simulink model "MTU_HVM_5_0a"  (Simulink 7.7)
settings: Solver=ode23  StartTime=0.0  StopTime=TEST_CYCLE(end,1)  FixedStep=0.01  RelTol=1e-3
InitFcn:
  | Vehicle_Init_File
values from neighbouring files (symbols this model uses):
  Batt_Aux_Load_W = 800    [Student_Design_Parameters.m]
  Engine_ACC_Loss_Nm = 4.6    [ICE_Tech_Specs.m]
  Engine_BSFC_2DMAP_g_kWh = Engine_BSFC_2DMAP_g_kWh'    [ICE_Tech_Specs.m]    (also in Student_Design_Parameters.m = 1.00*Engine_BSFC_2DMAP_g_kWh)
  Engine_Max_Speed_rpm = 6800    [ICE_Tech_Specs.m]
  Engine_Min_Speed_rpm = 600    [ICE_Tech_Specs.m]
  Engine_Startup_Fuel_g = 4.0*Engine_Displacement_L/3.6    (= 2.66666666667)    [ICE_Tech_Specs.m]
  Engine_Torque_2DMAP_Nm = Engine_Torque_2DMAP_Nm'    [ICE_Tech_Specs.m]
  Motor_Gear_Ratio = 1.00    (= 1)    [Student_Design_Parameters.m]
  Motor_Km = 0.94    [Motor_Tech_Specs.m]
  Motor_Ra = 0.106    [Motor_Tech_Specs.m]
  Motor_Torque_Peak_Nm = T    [Motor_Tech_Specs.m]
  Motor_Torque_Speed_Index_rpm = N    [Motor_Tech_Specs.m]
  TEST_CYCLE = [0 1 2 3 4 5 6 7 8 9 10 11 ... (1900 elements, 950x2)]    [Constant_Speed_Points_Cycle.mat]    (also in US06_Cycle.mat = [0 1 2 3 4 5 6 7 8 9 10 11 ... (1202 elements, 601x2)])
  TRANS_Differential_Ratio = 3.25    [Student_Design_Parameters.m]
  TRANS_DS_THRES = 1.0*TRANS_DS_THRES    [Student_Design_Parameters.m]
  TRANS_US_THRES = 1.0*TRANS_US_THRES    [Student_Design_Parameters.m]
  Vehicle_Drag_Coeff = F2/(0.5*Air_Density_kgm*Vehicle_Frontal_Area_m)    [Student_Design_Parameters.m]
  Vehicle_Frontal_Area_m = h*w*0.0254*0.0254    [Student_Design_Parameters.m]
  Vehicle_Mass_kg = 1549    [Student_Design_Parameters.m]
  Vehicle_Tire_Coeff_Rolling_Resistance = 0.008    [Student_Design_Parameters.m]
  Vehicle_Tire_Radius_m = 0.95*26.311/2*0.0254    (= 0.317442215)    [Student_Design_Parameters.m]
undefined symbols (not defined in the file or in its folder): Air_Density_kgm, Batt_a, Batt_Capacity_Ah, Batt_Const_V, Batt_dG, Batt_Disable_SOC, Batt_Initial_SOC, Batt_Lower_Volt_Limit_V, Batt_Max_Charge_Current_A, Batt_Max_Discharge_Current_A, Batt_Max_SOC, Batt_Min_SOC, Batt_Numb_Cells_N, Batt_OCV_Z, Batt_Resis_Ohms, Batt_Upper_Volt_Limit_V, Batt_Warburg_Capcitance_F, Batt_Warburg_Resis_Ohms, Fuel_Density_kgm3, Gravity, Max_Vehicle_Speed_Control_Error_mph, TRANS_Gear_Ratio, Vehicle_Tire_Rolling_Fric_Velocity_Modifier, Vehicle_Tire_Static_Fric_Coeff, Vehicle_Tractive_Force_Limit
libraries: simulink x8
(part 1 of 2)
settings Model: Creator=lawyerkm  LastModifiedBy=jnaber
settings SolverCC: ZeroCrossControl=DisableAll
settings OptimizationCC: InitFltsAndDblsToZero=on
settings DebuggingCC: AlgebraicLoopMsg=none  ArtificialAlgebraicLoopMsg=none  SaveWithParameterizedLinksMsg=none  SolverPrmCheckMsg=none  InheritedTsInSrcMsg=none  DiscreteInheritContinuousMsg=none  MultiTaskCondExecSysMsg=none  UnknownTsInhSupMsg=none  StrictBusMsg=None
settings HardwareCC: TargetHWDeviceType=32-bit Generic
settings SFSimCC: SimParseCustomCode=off
settings RTWCC: IncludeERTFirstTime=on
settings GRTTargetCC: TargetFcnLib=ansi_tfl_tmw.mat

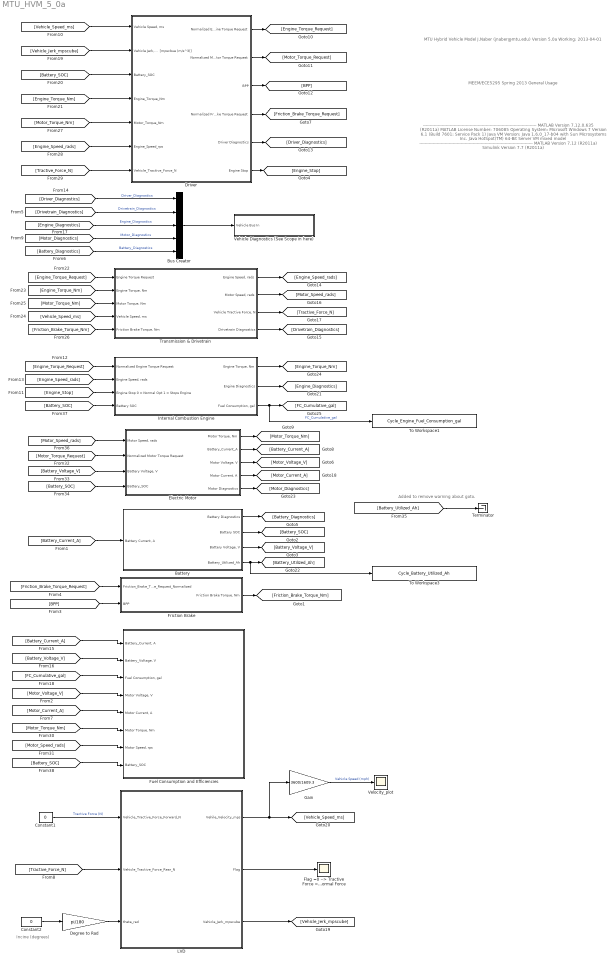
== system MTU_HVM_5_0a ==
  note: MTU Hybrid Vehicle Model
      | J.Naber (jnaber@mtu.edu)
      | Version 5.0a
      | Working:  2013-04-01
  note: MEEM/ECE5295
      | Spring 2013
      |
      | General Usage
  note: -------------------------------------------------------------------------------------
      | MATLAB Version 7.12.0.635 (R2011a)
      | MATLAB License Number: 706085
      | Operating System: Microsoft Windows 7 Version 6.1 (Build 7601: Service Pack 1)
      | Java VM Version: Java 1.6.0_17-b04 with Sun Microsystems Inc. Java HotSpot(TM) 64-Bit Server VM mixed model
      | -------------------------------------------------------------------------------------
      | MATLAB                                                Version 7.12       (R2011a)
      | Simulink                                                 Version 7.7        (R2011a)
  note: Added to remove warning about goto.
  note: Incine (degrees)
  Battery : Subsystem
  Bus Creator : BusCreator  Inputs=5
  Constant1 : Constant  Value=0
  Constant2 : Constant  Value=0
  Degree to Rad : Gain  Gain=pi/180
  Driver : Subsystem
  Electric Motor : Subsystem
  Flag =0 --> Tractive Force =< Road Friction * Normal Force Flag =1 --> Tractive Force > Road Friction * Normal Force : Scope
      settings: TimeRange=200  YMin=-1  YMax=1  SaveName=ScopeData2  SampleInput=on  SampleTime=0.5
  Friction Brake : Subsystem
  Fuel Consumption and Efficiencies : Subsystem
  Gain : Gain  Gain=3600/1609.3
  Internal Combustion Engine : Subsystem
  LVD : Subsystem
      mask help:
      | Vehicle of two axles riding on an incline. The aerodynamic parameters include the vehicle's frontal area and drag coefficient. The vehicle does not pitch or move vertically.
      |
      | The input signals Vehicle_Tractive_Force_Forward_N, Vehicle_Tractive_Force_Rear_N, and theta_rad specify the tractive force at forward and rear contact forces (N) and the incline angle (rad), respectively. The output signal Vehile_Velocity_mps, indicates the vehicle velocity (m/s).
      mask init:
      | g = 9.81;
      | rho = 1.2; %Air Density in kg/m^3
      mask Display:
      | port_label('input', 1, 'Vehicle_Tractive_Force_Front_N')
      | port_label('input', 2, 'Vehicle_Tractive_Force_Rear_N')
      | port_label('input', 3, 'theta_rad')
      | port_label('output', 1, 'Vehile_Velocity_mps')
      | port_label('output', 2, 'Flag')
      | port_label('output', 3, 'Vehicle_Jerk_mpscube')
  Terminator : Terminator
  To Workspace1 : ToWorkspace  VariableName=Cycle_Engine_Fuel_Consumption_gal  SampleTime=-1  SaveFormat=Array
      settings: MaxDataPoints=1
  To Workspace3 : ToWorkspace  VariableName=Cycle_Battery_Utilized_Ah  SampleTime=-1  SaveFormat=Array
      settings: MaxDataPoints=1
  Transmission & Drivetrain : Subsystem
  Vehicle Diagnostics (See Scope in here) : Subsystem
  Velocity_plot : Scope
      settings: TimeRange=200  YMax=60  SaveName=Vehicle_Speed  SampleTime=0.5
  wires:
  Driver/2(Normalized Motor Torque Request) -> [Motor_Torque_Request]
  Driver/1(Normalized Engine Torque Request) -> [Engine_Torque_Request]
  Driver/3(BPP) -> [BPP]
  Driver/5(Driver Diagnostics) -> [Driver_Diagnostics]
  [Vehicle_Speed_ms] -> Driver/1("Vehicle Speed, ms")
  [Driver_Diagnostics] -> Bus Creator/1  "Driver_Diagnostics"
  [Drivetrain_Diagnostics] -> Bus Creator/2  "Drivetrain_Diagnostics"
  Bus Creator/1 -> Vehicle Diagnostics (See Scope in here)/1(Vehicle Bus In)
  [Motor_Diagnostics] -> Bus Creator/4  "Motor_Diagnostics"
  [Battery_Diagnostics] -> Bus Creator/5  "Battery_Diagnostics"
  [Engine_Diagnostics] -> Bus Creator/3  "Engine_Diagnostics"
  LVD/1(Vehile_Velocity_mps) -> Gain/1, [Vehicle_Speed_ms]
  Constant1/1 -> LVD/1(Vehicle_Tractive_Force_Forward_N)  "Tractive Force (N)"
  Constant2/1 -> Degree to Rad/1
  Gain/1 -> Velocity_plot/1  "Vehicle Speed (mph)"
  LVD/2(Flag) -> Flag =0 --> Tractive Force =< Road Friction * Normal Force Flag =1 --> Tractive Force > Road Friction * Normal Force/1
  [Tractive_Force_N] -> LVD/2(Vehicle_Tractive_Force_Rear_N)
  [Battery_Current_A] -> Fuel Consumption and Efficiencies/1("Battery_Current, A")
  [FC_Cumulative_gal] -> Fuel Consumption and Efficiencies/3("Fuel Consumption, gal")
  [Battery_Voltage_V] -> Fuel Consumption and Efficiencies/2("Battery_Voltage, V")
  [Motor_Voltage_V] -> Fuel Consumption and Efficiencies/4("Motor Voltage, V")
  [Motor_Current_A] -> Fuel Consumption and Efficiencies/5("Motor Current, A")
  [Motor_Torque_Nm] -> Fuel Consumption and Efficiencies/6("Motor Torque, Nm")
  [Motor_Speed_rads] -> Fuel Consumption and Efficiencies/7("Motor Speed, rps")
  Transmission & Drivetrain/4(Drivetrain Diagnostics) -> [Drivetrain_Diagnostics]
  Transmission & Drivetrain/1("Engine Speed, rads") -> [Engine_Speed_rads]
  Transmission & Drivetrain/2("Motor Speed, rads") -> [Motor_Speed_rads]
  Transmission & Drivetrain/3("Vehicle Tractive Force, N") -> [Tractive_Force_N]
  [Engine_Torque_Request] -> Transmission & Drivetrain/1(Engine Torque Request)
  [Engine_Torque_Nm] -> Transmission & Drivetrain/2("Engine Torque, Nm")
  [Motor_Torque_Nm] -> Transmission & Drivetrain/3("Motor Torque, Nm")
  [Vehicle_Speed_ms] -> Transmission & Drivetrain/4("Vehicle Speed, ms")
  [Friction_Brake_Torque_Nm] -> Transmission & Drivetrain/5("Friction Brake Torque, Nm")
  [Motor_Speed_rads] -> Electric Motor/1("Motor Speed, rads")
  [Motor_Torque_Request] -> Electric Motor/2(Normalized Motor Torque Request)
  [Battery_Voltage_V] -> Electric Motor/3("Battery Voltage, V")
  Electric Motor/1("Motor Torque, Nm") -> [Motor_Torque_Nm]
  [Battery_SOC] -> Electric Motor/4(Battery_SOC)
  Driver/4(Normalized Friction Brake Torque Request) -> [Friction_Brake_Torque_Request]
  [BPP] -> Friction Brake/2(BPP)
  [Friction_Brake_Torque_Request] -> Friction Brake/1(Friction_Brake_Torque_Request_Normalized)
  Friction Brake/1("Friction Brake Torque, Nm") -> [Friction_Brake_Torque_Nm]
  Electric Motor/2(Battery_Current_A) -> [Battery_Current_A]
  Electric Motor/3("Motor Voltage, V") -> [Motor_Voltage_V]
  Electric Motor/4("Motor Current, A") -> [Motor_Current_A]
  Internal Combustion Engine/2(Engine Diagnostics) -> [Engine_Diagnostics]
  Internal Combustion Engine/1("Engine Torque, Nm") -> [Engine_Torque_Nm]
  [Engine_Torque_Request] -> Internal Combustion Engine/1(Normalized Engine Torque Request)
  [Engine_Speed_rads] -> Internal Combustion Engine/2("Engine Speed, rads")
  Internal Combustion Engine/3("Fuel Consumption, gal") -> [FC_Cumulative_gal], To Workspace1/1  "FC_Cumulative_gal"
  [Engine_Stop] -> Internal Combustion Engine/3(Engine Stop 0 = Normal Opt 1 = Stops Engine)
  Driver/6(Engine Stop) -> [Engine_Stop]
  LVD/3(Vehicle_Jerk_mpscube) -> [Vehicle_Jerk_mpscube]
  [Vehicle_Jerk_mpscube] -> Driver/2("Vehicle Jerk,  [mpscbue (m/s^3)]")
  Electric Motor/5(Motor Diagnostics) -> [Motor_Diagnostics]
  [Battery_SOC] -> Driver/3(Battery_SOC)
  [Engine_Torque_Nm] -> Driver/4(Engine_Torque_Nm)
  [Motor_Torque_Nm] -> Driver/5(Motor_Torque_Nm)
  [Engine_Speed_rads] -> Driver/6(Engine_Speed_rps)
  [Tractive_Force_N] -> Driver/7(Vehicle_Tractive_Force_N)
  [Battery_Utilized_Ah] -> Terminator/1
  [Battery_Current_A] -> Battery/1("Battery Current, A")
  Battery/1(Battery Diagnostics) -> [Battery_Diagnostics]
  [Battery_SOC] -> Internal Combustion Engine/4(Battery SOC)
  Battery/3("Battery Voltage, V") -> [Battery_Voltage_V]
  Battery/2(Battery SOC) -> [Battery_SOC]
  Battery/4(Battery_Utilized_Ah) -> [Battery_Utilized_Ah], To Workspace3/1
  [Battery_SOC] -> Fuel Consumption and Efficiencies/8("Battery_SOC ")
  Degree to Rad/1 -> LVD/3(theta_rad)

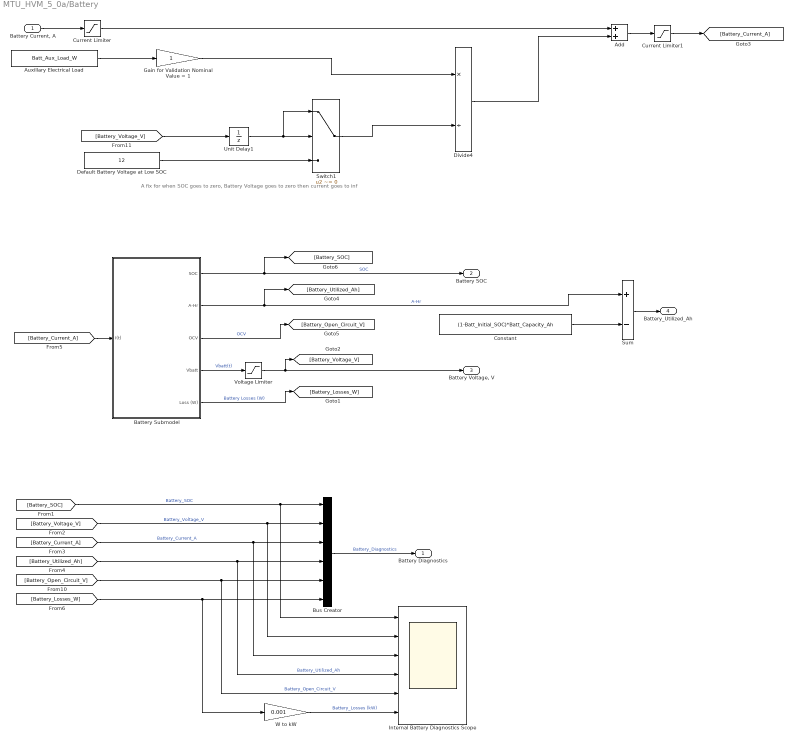
== system MTU_HVM_5_0a/Battery ==
  note: A fix for when SOC goes to zero,
      |  Battery Voltage goes to zero then current goes to inf
  "Battery Current, A" : Inport
  Add : Sum
  Auxillary Electrical Load : Constant  Value=Batt_Aux_Load_W
  Battery Submodel : Subsystem  mask{Vo=Batt_Const_V, Rbatt=Batt_Resis_Ohms, Cd=Batt_Warburg_Capcitance_F, Rd=Batt_Warburg_Resis_Ohms, Q=Batt_Capacity_Ah, dG=Batt_dG, a=Batt_a, SOC_Init=Batt_Initial_SOC, Batt_Numb_Cells_N=Batt_Numb_Cells_N, Batt_OCV_Z=Batt_OCV_Z}
      mask prompts: Vo "Fully Charged Voltage Vo (V)"; Rbatt "Battery Resistance Rc (Ohm)"; Cd "Warburg Capacitance Cd (F)"; Rd "Warburg Resistance Rd (Ohm)"; Q "Amp Hour Capacity  Q (A-Hr)"; dG "Free energy difference dG"; a "Molecular interaction exponent a"; SOC_Init "State of Charge Initial (-)"; Batt_Numb_Cells_N "Number of Cells"; Batt_OCV_Z "Z Parameter"
      mask help:
      | Lithium Cobalt Oxide/Carbon
      |     dG = -355000,   a = 4
      |
      | Nickel Metal Hydride
      |     dG = -115000,   a=0.8
  Bus Creator : BusCreator  Inputs=6
  Constant : Constant  Value=(1-Batt_Initial_SOC)*Batt_Capacity_Ah  SampleTime=-1
  Current Limiter : Saturate  UpperLimit=Batt_Max_Charge_Current_A  LowerLimit=Batt_Max_Discharge_Current_A
  Current Limiter1 : Saturate  UpperLimit=Batt_Max_Charge_Current_A  LowerLimit=Batt_Max_Discharge_Current_A
  Default Battery Voltage at Low SOC : Constant  Value=12  SampleTime=-1
  Divide4 : Product  Inputs=*/
  Gain for Validation Nominal Value = 1 : Gain
  Internal Battery Diagnostics Scope : Scope  NumInputPorts=6
      settings: TimeRange=1000  YMin=5.55112e-017~62.75~71.25~0.5~90~2.75  YMax=0.8~64.25~78.75~5~102~4.25  SaveName=Diagnostics_Battery  SampleInput=on  SampleTime=0.1
  Sum : Sum  Inputs=+-
  Switch1 : Switch  Criteria=u2 ~= 0  Threshold=12
  Unit Delay1 : UnitDelay  X0=Batt_Const_V  SampleTime=-1
  Voltage Limiter : Saturate  UpperLimit=Batt_Upper_Volt_Limit_V  LowerLimit=Batt_Lower_Volt_Limit_V  LinearizeAsGain=off
  W to kW : Gain  Gain=0.001
  Battery Diagnostics : Outport
  Battery SOC : Outport  Port=2
  "Battery Voltage, V" : Outport  Port=3
  Battery_Utilized_Ah : Outport  Port=4
  wires:
  Bus Creator/1 -> Battery Diagnostics/1  "Battery_Diagnostics"
  [Battery_SOC] -> Bus Creator/1, Internal Battery Diagnostics Scope/1  "Battery_SOC"
  [Battery_Voltage_V] -> Bus Creator/2, Internal Battery Diagnostics Scope/2  "Battery_Voltage_V"
  [Battery_Current_A] -> Bus Creator/3, Internal Battery Diagnostics Scope/3  "Battery_Current_A"
  "Battery Current, A"/1 -> Current Limiter/1
  [Battery_Utilized_Ah] -> Bus Creator/4, Internal Battery Diagnostics Scope/4  "Battery_Utilized_Ah"
  [Battery_Open_Circuit_V] -> Bus Creator/5, Internal Battery Diagnostics Scope/5  "Battery_Open_Circuit_V"
  Add/1 -> Current Limiter1/1
  Auxillary Electrical Load/1 -> Gain for Validation Nominal Value = 1/1
  [Battery_Losses_W] -> Bus Creator/6, W to kW/1
  Default Battery Voltage at Low SOC/1 -> Switch1/3
  [Battery_Voltage_V] -> Unit Delay1/1
  W to kW/1 -> Internal Battery Diagnostics Scope/6  "Battery_Losses (kW)"
  Switch1/1 -> Divide4/2
  Unit Delay1/1 -> Switch1/1, Switch1/2
  Battery Submodel/1(SOC) -> [Battery_SOC], Battery SOC/1  "SOC"
  Battery Submodel/2(A-Hr) -> [Battery_Utilized_Ah], Sum/1  "A-Hr"
  Battery Submodel/3(OCV) -> [Battery_Open_Circuit_V]  "OCV"
  Battery Submodel/5(Loss (W)) -> [Battery_Losses_W]  "Battery Losses (W)"
  Battery Submodel/4(Vbatt) -> Voltage Limiter/1  "Vbatt(t)"
  [Battery_Current_A] -> Battery Submodel/1(I(t))
  Divide4/1 -> Add/2
  Gain for Validation Nominal Value = 1/1 -> Divide4/1
  Current Limiter1/1 -> [Battery_Current_A]
  Current Limiter/1 -> Add/1
  Voltage Limiter/1 -> [Battery_Voltage_V], "Battery Voltage, V"/1
  Sum/1 -> Battery_Utilized_Ah/1
  Constant/1 -> Sum/2

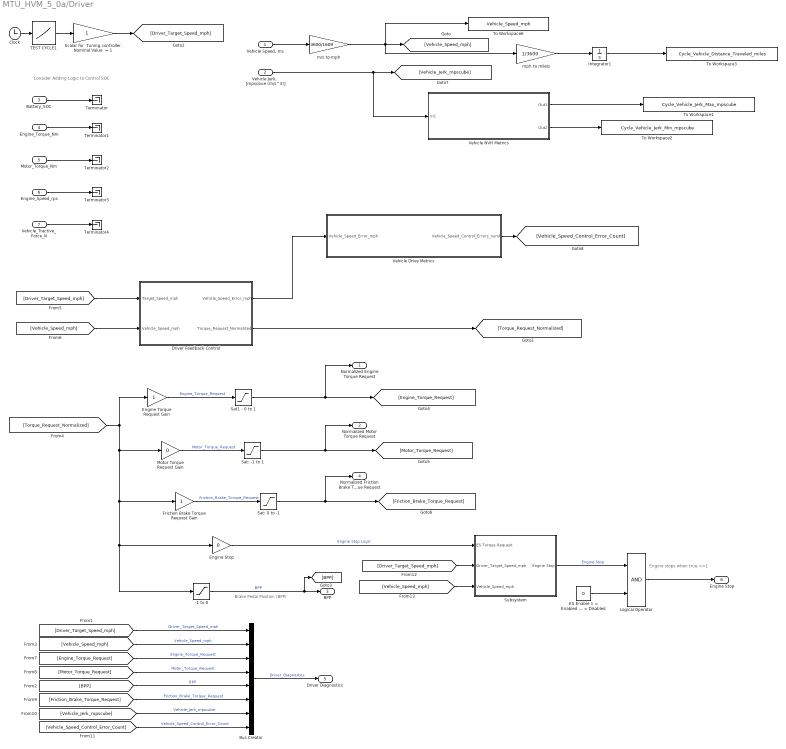
== system MTU_HVM_5_0a/Driver ==
  note: Consider Adding Logic to Control SOC
  note: Brake Pedal Position
      |
      | (BPP)
  note: Engine stops when
      |
      | true ==1
  "Vehicle Speed, ms" : Inport
  "Vehicle Jerk,  [mpscbue (m/s^3)]" : Inport  Port=2
  Battery_SOC : Inport  Port=3
  Engine_Torque_Nm : Inport  Port=4
  Motor_Torque_Nm : Inport  Port=5
  Engine_Speed_rps : Inport  Port=6
  Vehicle_Tractive_Force_N : Inport  Port=7
  -1 to 0 : Saturate  UpperLimit=0  LowerLimit=-1
  Bus Creator : BusCreator  Inputs=8
  Clock : Clock
      settings: Decimation=10
  Driver Feedback Control : Subsystem
  ES Enable 1 = Enabled 0 = Disabled : Constant  Value=0  SampleTime=-1
  "Engine Stop " : Gain  Gain=0
  Engine Torque Request Gain : Gain
  Friction Brake Torque Request Gain : Gain
  Integrator1 : Integrator
  Logical Operator : Logic  AllPortsSameDT=off  OutDataTypeStr=boolean
  Motor Torque Request Gain : Gain  Gain=0
  Sat1 - 0 to 1 : Saturate  UpperLimit=1  LowerLimit=0
  Sat: -1 to 1 : Saturate  UpperLimit=1  LowerLimit=-1
  Sat: 0 to -1 : Saturate  UpperLimit=0  LowerLimit=-1
  Scalar for  Tuning controller. Nominal Value  = 1 : Gain
  Subsystem : Subsystem
  TEST CYCLE1 : Lookup  InputValues=TEST_CYCLE(:,1)  Table=TEST_CYCLE(:,2)  LookUpMeth=Interpolation-Use End Values
  Terminator{,1..4} (5 alike) : Terminator
  To Workspace1 : ToWorkspace  VariableName=Cycle_Vehicle_Jerk_Max_mpscube  SampleTime=-1  SaveFormat=Array
      settings: MaxDataPoints=1
  To Workspace2 : ToWorkspace  VariableName=Cycle_Vehicle_Jerk_Min_mpscube  SampleTime=-1  SaveFormat=Array
      settings: MaxDataPoints=1
  To Workspace3 : ToWorkspace  VariableName=Cycle_Vehicle_Distance_Traveled_miles  SampleTime=-1  SaveFormat=Array
      settings: MaxDataPoints=1
  To Workspace6 : ToWorkspace  VariableName=Vehicle_Speed_mph  SampleTime=-1  SaveFormat=Array
      settings: MaxDataPoints=1
  Vehicle Drive Metrics : Subsystem
  Vehicle NVH Metrics : Subsystem
  m/s to mph : Gain  Gain=3600/1609
  mph to mile/s : Gain  Gain=1/3600
  Normalized Engine Torque Request : Outport
  Normalized Motor Torque Request : Outport  Port=2
  BPP : Outport  Port=3
  Normalized Friction Brake Torque Request : Outport  Port=4
  Driver Diagnostics : Outport  Port=5
  Engine Stop : Outport  Port=6
  wires:
  [Vehicle_Speed_mph] -> Bus Creator/2  "Vehicle_Speed_mph"
  Bus Creator/1 -> Driver Diagnostics/1  "Driver_Diagnostics"
  Clock/1 -> TEST CYCLE1/1
  [Driver_Target_Speed_mph] -> Driver Feedback Control/1(Target_Speed_mph)
  Driver Feedback Control/2(Torque_Request_Normalized) -> [Torque_Request_Normalized]
  "Vehicle Speed, ms"/1 -> m/s to mph/1
  m/s to mph/1 -> [Vehicle_Speed_mph], mph to mile/s/1, To Workspace6/1
  [Torque_Request_Normalized] -> Engine Torque Request Gain/1, Motor Torque Request Gain/1, Friction Brake Torque Request Gain/1, -1 to 0/1, "Engine Stop "/1
  [Motor_Torque_Request] -> Bus Creator/4  "Motor_Torque_Request"
  [Engine_Torque_Request] -> Bus Creator/3  "Engine_Torque_Request"
  -1 to 0/1 -> [BPP], BPP/1  "BPP"
  Motor Torque Request Gain/1 -> Sat: -1 to 1/1  "Motor_Torque_Request"
  Engine Torque Request Gain/1 -> Sat1 - 0 to 1/1  "Engine_Torque_Request"
  Sat1 - 0 to 1/1 -> [Engine_Torque_Request], Normalized Engine Torque Request/1
  TEST CYCLE1/1 -> Scalar for  Tuning controller. Nominal Value  = 1/1
  Friction Brake Torque Request Gain/1 -> Sat: 0 to -1/1  "Friction_Brake_Torque_Request"
  Sat: -1 to 1/1 -> Normalized Motor Torque Request/1, [Motor_Torque_Request]
  Sat: 0 to -1/1 -> Normalized Friction Brake Torque Request/1, [Friction_Brake_Torque_Request]
  "Engine Stop "/1 -> Subsystem/1(ES Torque Request)  "Engine Stop Logic"
  "Vehicle Jerk,  [mpscbue (m/s^3)]"/1 -> [Vehicle_Jerk_mpscube], Vehicle NVH Metrics/1(In1)
  [Driver_Target_Speed_mph] -> Bus Creator/1  "Driver_Target_Speed_mph"
  [BPP] -> Bus Creator/5  "BPP"
  [Friction_Brake_Torque_Request] -> Bus Creator/6  "Friction_Brake_Torque_Request"
  [Vehicle_Jerk_mpscube] -> Bus Creator/7  "Vehicle_Jerk_mpscube"
  Vehicle NVH Metrics/1(Out1) -> To Workspace1/1
  Vehicle NVH Metrics/2(Out2) -> To Workspace2/1
  mph to mile/s/1 -> Integrator1/1
  Integrator1/1 -> To Workspace3/1
  [Vehicle_Speed_Control_Error_Count] -> Bus Creator/8  "Vehicle_Speed_Control_Error_Count"
  Battery_SOC/1 -> Terminator/1
  Engine_Torque_Nm/1 -> Terminator1/1
  Motor_Torque_Nm/1 -> Terminator2/1
  Engine_Speed_rps/1 -> Terminator3/1
  Vehicle_Tractive_Force_N/1 -> Terminator4/1
  Scalar for  Tuning controller. Nominal Value  = 1/1 -> [Driver_Target_Speed_mph]
  Vehicle Drive Metrics/1(Vehicle_Speed_Control_Errors_numb) -> [Vehicle_Speed_Control_Error_Count]
  [Driver_Target_Speed_mph] -> Subsystem/2(Driver_Target_Speed_mph)
  [Vehicle_Speed_mph] -> Subsystem/3(Vehicle_Speed_mph)
  Subsystem/1(Engine Stop) -> Logical Operator/1  "Engine Stop"
  Logical Operator/1 -> Engine Stop/1
  ES Enable 1 = Enabled 0 = Disabled/1 -> Logical Operator/2
  Driver Feedback Control/1(Vehicle_Speed_Error_mph) -> Vehicle Drive Metrics/1(Vehicle_Speed_Error_mph)
  [Vehicle_Speed_mph] -> Driver Feedback Control/2(Vehicle_Speed_mph)

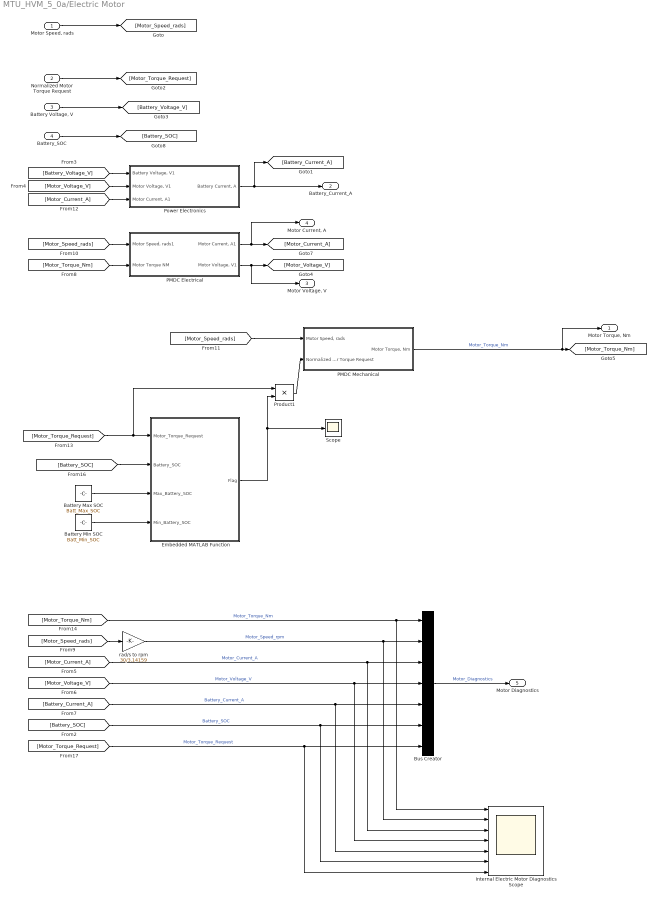
== system MTU_HVM_5_0a/Electric Motor ==
  "Motor Speed, rads" : Inport
  Normalized Motor Torque Request : Inport  Port=2
  "Battery Voltage, V" : Inport  Port=3
  Battery_SOC : Inport  Port=4
  Battery Max SOC : Constant  Value=Batt_Max_SOC
  Battery Min SOC : Constant  Value=Batt_Min_SOC
  Bus Creator : BusCreator  Inputs=7
  Embedded MATLAB Function : Stateflow chart  TreatAsAtomicUnit=on
  Internal Electric Motor Diagnostics Scope : Scope  NumInputPorts=7
      settings: YMin=-50~-100~-50~-25~-10~0.85~-0.75  YMax=300~800~250~125~90~0.9~1  SaveName=Diagnostics_EMachine  SampleInput=on  SampleTime=0.1
  PMDC Electrical : Subsystem
  PMDC Mechanical : Subsystem
  Power Electronics : Subsystem
  Product1 : Product  RndMeth=Zero
  Scope : Scope
      settings: YMin=0  YMax=1  SaveName=ScopeData9  SampleInput=on  SampleTime=0.5
  rad/s to rpm : Gain  Gain=30/3.14159
  "Motor Torque, Nm" : Outport
  Battery_Current_A : Outport  Port=2
  "Motor Voltage, V" : Outport  Port=3
  "Motor Current, A" : Outport  Port=4
  Motor Diagnostics : Outport  Port=5
  wires:
  "Motor Speed, rads"/1 -> [Motor_Speed_rads]
  [Motor_Speed_rads] -> PMDC Electrical/1("Motor Speed, rads1")
  PMDC Electrical/1("Motor Current, A1") -> [Motor_Current_A], "Motor Current, A"/1
  [Motor_Speed_rads] -> PMDC Mechanical/1("Motor Speed, rads")
  Normalized Motor Torque Request/1 -> [Motor_Torque_Request]
  "Battery Voltage, V"/1 -> [Battery_Voltage_V]
  PMDC Mechanical/1("Motor Torque, Nm") -> [Motor_Torque_Nm], "Motor Torque, Nm"/1  "Motor_Torque_Nm"
  [Motor_Torque_Nm] -> PMDC Electrical/2(Motor Torque NM)
  Power Electronics/1("Battery Current, A") -> Battery_Current_A/1, [Battery_Current_A]
  [Battery_Voltage_V] -> Power Electronics/1("Battery Voltage, V1")
  [Motor_Current_A] -> Power Electronics/3("Motor Current, A1")
  PMDC Electrical/2("Motor Voltage, V1") -> [Motor_Voltage_V], "Motor Voltage, V"/1
  [Motor_Voltage_V] -> Power Electronics/2("Motor Voltage, V1")
  Battery_SOC/1 -> [Battery_SOC]
  Product1/1 -> PMDC Mechanical/2(Normalized Motor Torque Request)
  [Motor_Torque_Request] -> Embedded MATLAB Function/1(Motor_Torque_Request), Product1/1
  [Battery_SOC] -> Embedded MATLAB Function/2(Battery_SOC)
  Battery Min SOC/1 -> Embedded MATLAB Function/4(Min_Battery_SOC)
  Battery Max SOC/1 -> Embedded MATLAB Function/3(Max_Battery_SOC)
  Embedded MATLAB Function/1(Flag) -> Product1/2, Scope/1
  Bus Creator/1 -> Motor Diagnostics/1  "Motor_Diagnostics"
  [Motor_Torque_Nm] -> Bus Creator/1, Internal Electric Motor Diagnostics Scope/1  "Motor_Torque_Nm"
  [Motor_Speed_rads] -> rad/s to rpm/1
  [Motor_Current_A] -> Bus Creator/3, Internal Electric Motor Diagnostics Scope/3  "Motor_Current_A"
  [Motor_Voltage_V] -> Bus Creator/4, Internal Electric Motor Diagnostics Scope/4  "Motor_Voltage_V"
  rad/s to rpm/1 -> Bus Creator/2, Internal Electric Motor Diagnostics Scope/2  "Motor_Speed_rpm"
  [Battery_Current_A] -> Bus Creator/5, Internal Electric Motor Diagnostics Scope/5  "Battery_Current_A"
  [Battery_SOC] -> Bus Creator/6, Internal Electric Motor Diagnostics Scope/6  "Battery_SOC"
  [Motor_Torque_Request] -> Bus Creator/7, Internal Electric Motor Diagnostics Scope/7  "Motor_Torque_Request"

== system MTU_HVM_5_0a/Friction Brake ==
  Friction_Brake_Torque_Request_Normalized : Inport
  BPP : Inport  Port=2
  Coeff of friction : Constant  Value=Vehicle_Tire_Static_Fric_Coeff
  Compare To Zero : simulink/Logic and Bit Operations/Compare To Zero  SystemSampleTime=-1  relop=<  LogicOutDataTypeMode=uint8  ZeroCross=off
  Product : Product  Inputs=4  RndMeth=Zero
  Product1 : Product  RndMeth=Zero
  "Vehicle Normal Force, N" : Constant  Value=(Vehicle_Mass_kg*Gravity)/2
  "Wheel Radius, m" : Constant  Value=Vehicle_Tire_Radius_m
  "Friction Brake Torque, Nm" : Outport
  wires:
  Friction_Brake_Torque_Request_Normalized/1 -> Product/1
  "Wheel Radius, m"/1 -> Product/2
  Coeff of friction/1 -> Product/3
  Product/1 -> Product1/1
  "Vehicle Normal Force, N"/1 -> Product/4
  BPP/1 -> Compare To Zero/1
  Compare To Zero/1 -> Product1/2
  Product1/1 -> "Friction Brake Torque, Nm"/1

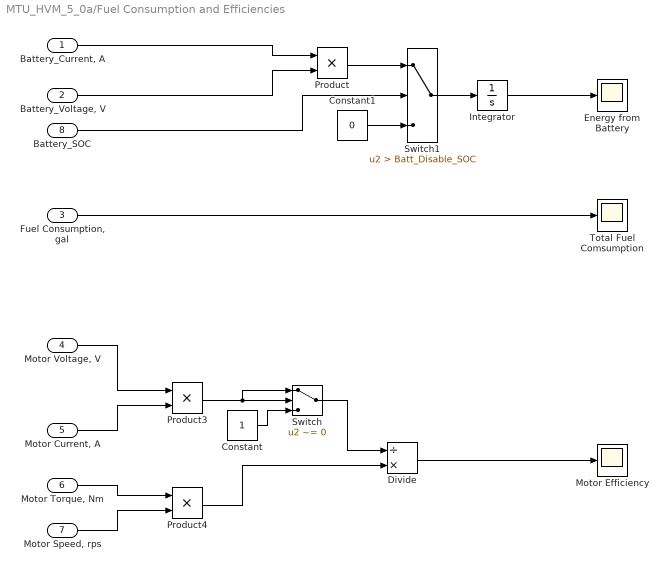
== system MTU_HVM_5_0a/Fuel Consumption and Efficiencies ==
  "Battery_Current, A" : Inport
  "Battery_Voltage, V" : Inport  Port=2
  "Fuel Consumption, gal" : Inport  Port=3
  "Motor Voltage, V" : Inport  Port=4
  "Motor Current, A" : Inport  Port=5
  "Motor Torque, Nm" : Inport  Port=6
  "Motor Speed, rps" : Inport  Port=7
  "Battery_SOC " : Inport  Port=8
  Constant : Constant
  Constant1 : Constant  Value=0
  Divide : Product  Inputs=/*
  Energy from Battery : Scope
      settings: YMin=0  YMax=180  SaveName=ScopeData11  SampleInput=on  SampleTime=0.5
  Integrator : Integrator
  Motor Efficiency : Scope
      settings: YMin=-225  YMax=300  SaveName=ScopeData12  SampleInput=on  SampleTime=0.5
  Product : Product  RndMeth=Zero
  Product3 : Product  RndMeth=Zero
  Product4 : Product  RndMeth=Zero
  Switch : Switch  Criteria=u2 ~= 0
  Switch1 : Switch  Criteria=u2 > Threshold  Threshold=Batt_Disable_SOC
  Total Fuel Comsumption : Scope
      settings: SaveName=ScopeData25  SampleInput=on  SampleTime=0.5
  wires:
  "Battery_Current, A"/1 -> Product/1
  "Battery_Voltage, V"/1 -> Product/2
  Integrator/1 -> Energy from Battery/1
  "Motor Voltage, V"/1 -> Product3/1
  "Motor Current, A"/1 -> Product3/2
  "Motor Torque, Nm"/1 -> Product4/1
  "Motor Speed, rps"/1 -> Product4/2
  Product4/1 -> Divide/2
  Divide/1 -> Motor Efficiency/1
  "Fuel Consumption, gal"/1 -> Total Fuel Comsumption/1
  Product3/1 -> Switch/2, Switch/1
  Switch/1 -> Divide/1
  Constant/1 -> Switch/3
  "Battery_SOC "/1 -> Switch1/2
  Constant1/1 -> Switch1/3
  Switch1/1 -> Integrator/1
  Product/1 -> Switch1/1

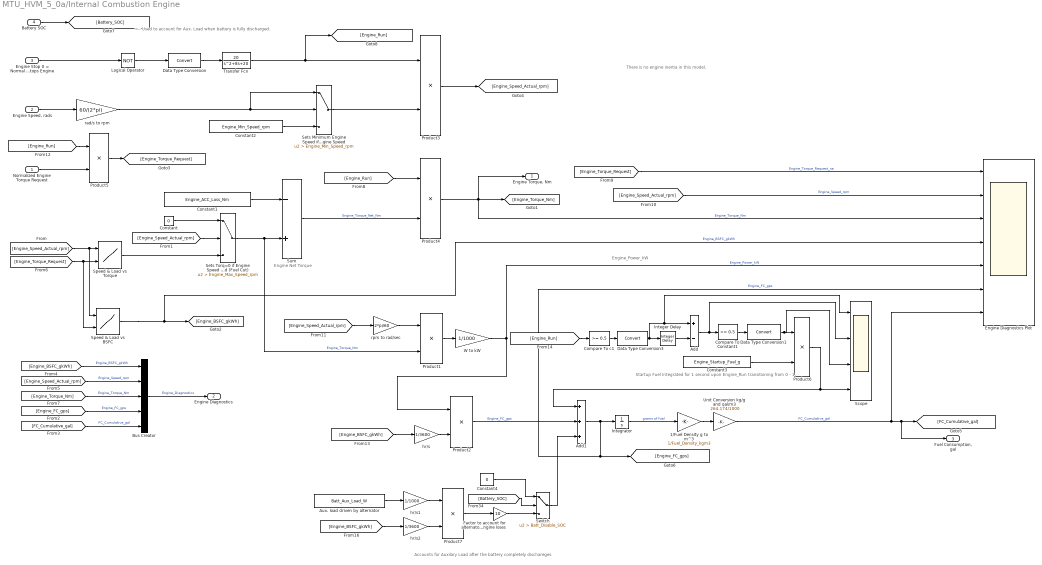
== system MTU_HVM_5_0a/Internal Combustion Engine ==
  note: Engine
      | Net Torque
  note: There is no engine inertia in this model.
  note: Startup Fuel
      | Integrated for 1 second upon Engine_Run transitioning from 0 - 1.
  note: Engine_Power_kW
  note: <-- Used to account for Aux. Load when battery
      | is fully discharged.
  note: Accounts for Auxilary Load after
      | the battery completely dischareges
  Normalized Engine Torque Request : Inport
  "Engine Speed, rads" : Inport  Port=2
  Engine Stop 0 = Normal Opt 1 = Stops Engine : Inport  Port=3
  Battery SOC : Inport  Port=4
  1/Fuel Density g to m^3 : Gain  Gain=1/Fuel_Density_kgm3
  Add : Sum  Inputs=+-
  Add1 : Sum  Inputs=+++
  Aux. load driven by alternator : Constant  Value=Batt_Aux_Load_W
  Bus Creator : BusCreator  Inputs=5
  Compare To Constant1 : simulink/Logic and Bit Operations/Compare To Constant  SystemSampleTime=-1  relop=>=  const=0.5  LogicOutDataTypeMode=uint8  ZeroCross=off
  Compare To c1 : simulink/Logic and Bit Operations/Compare To Constant  SystemSampleTime=-1  relop=>=  const=0.5  LogicOutDataTypeMode=uint8  ZeroCross=off
  Constant : Constant  Value=0
  Constant1 : Constant  Value=Engine_ACC_Loss_Nm
  Constant2 : Constant  Value=Engine_Min_Speed_rpm
  Constant3 : Constant  Value=Engine_Startup_Fuel_g  SampleTime=-1
  Constant4 : Constant  Value=0
  Data Type Conversion : DataTypeConversion
  Data Type Conversion1 : DataTypeConversion
  Data Type Conversion3 : DataTypeConversion
  Engine Diagnostics Plot : Scope  NumInputPorts=7
      settings: YMin=0~0~40~-50~-5~0~0  YMax=0.9~2500~120~3000~50~3.5~1  SaveName=Diagnostics_Engine  SampleInput=on  SampleTime=0.1
  Factor to account for  alternator and engine loses : Gain  Gain=10
  Integer Delay : simulink/Discrete/Integer Delay  NumDelays=10  InputProcessing=Inherited  vinit=0.0  samptime=0.1
  Integrator : Integrator
  Logical Operator : Logic  Operator=NOT  AllPortsSameDT=off  OutDataTypeStr=boolean
  Product{1..7} (7 alike) : Product  SaturateOnIntegerOverflow=on  OutDataTypeStr=Inherit: Same as first input
  Scope : Scope  NumInputPorts=4
      settings: YMin=-5~-5~-2~0  YMax=5~5~15~10  SaveName=ScopeData4  SampleInput=on  SampleTime=1
  Sets Minimum Engine Speed if Engine Speed > Min Engine Speed : Switch  Criteria=u2 > Threshold  Threshold=Engine_Min_Speed_rpm
  Sets Torq=0 if Engine Speed > Max Engine Speed (Fuel Cut) : Switch  Criteria=u2 > Threshold  Threshold=Engine_Max_Speed_rpm  ZeroCross=off
  Speed & Load vs BSFC : Lookup2D  RowIndex=Engine_2DMAP_Index_RPM  ColumnIndex=Engine_2DMAP_Index_TR  Table=Engine_BSFC_2DMAP_g_kWh  LookUpMeth=Interpolation-Use End Values
  Speed & Load vs Torque : Lookup2D  RowIndex=Engine_2DMAP_Index_RPM  ColumnIndex=Engine_2DMAP_Index_TR  Table=Engine_Torque_2DMAP_Nm  LookUpMeth=Interpolation-Use End Values
  Sum : Sum  Inputs=-+
  Switch : Switch  Criteria=u2 > Threshold  Threshold=Batt_Disable_SOC
  Transfer Fcn : TransferFcn  Numerator=20  Denominator=[1 8 20]
  Unit Conversion kg/g and gal/m3 : Gain  Gain=264.174/1000
  W to kW : Gain  Gain=1/1000
  hr/s : Gain  Gain=1/3600
  hr/s1 : Gain  Gain=1/1000
  hr/s2 : Gain  Gain=1/3600
  rad/s to rpm : Gain  Gain=60/(2*pi)
  rpm to rad/sec : Gain  Gain=2*pi/60
  "Engine Torque, Nm" : Outport
  Engine Diagnostics : Outport  Port=2
  "Fuel Consumption, gal" : Outport  Port=3
  wires:
  Constant/1 -> Sets Torq=0 if Engine Speed > Max Engine Speed (Fuel Cut)/1
  Speed & Load vs Torque/1 -> Sets Torq=0 if Engine Speed > Max Engine Speed (Fuel Cut)/3
  "Engine Speed, rads"/1 -> rad/s to rpm/1
  [Engine_Speed_Actual_rpm] -> Sets Torq=0 if Engine Speed > Max Engine Speed (Fuel Cut)/2
  Speed & Load vs BSFC/1 -> [Engine_BSFC_gkWh], Engine Diagnostics Plot/4  "Engine_BSFC_gkWh"
  Bus Creator/1 -> Engine Diagnostics/1  "Engine_Diagnostics"
  [Engine_BSFC_gkWh] -> Bus Creator/1  "Engine_BSFC_gkWh"
  [Engine_Speed_Actual_rpm] -> Bus Creator/2  "Engine_Speed_rpm"
  [Engine_Torque_Nm] -> Bus Creator/3  "Engine_Torque_Nm"
  rad/s to rpm/1 -> Sets Minimum Engine Speed if Engine Speed > Min Engine Speed/2, Sets Minimum Engine Speed if Engine Speed > Min Engine Speed/1
  [Engine_Speed_Actual_rpm] -> Speed & Load vs Torque/1, Speed & Load vs BSFC/1
  [Engine_Torque_Request] -> Speed & Load vs Torque/2, Speed & Load vs BSFC/2
  [Engine_Torque_Request] -> Engine Diagnostics Plot/1  "Engine_Torque_Request_na"
  [Engine_Speed_Actual_rpm] -> Engine Diagnostics Plot/2  "Engine_Speed_rpm"
  [Engine_Speed_Actual_rpm] -> rpm to rad/sec/1
  rpm to rad/sec/1 -> Product1/1
  Product1/1 -> W to kW/1
  W to kW/1 -> Engine Diagnostics Plot/5, Product2/1  "Engine_Power_kW"
  [Engine_BSFC_gkWh] -> hr/s/1
  Product2/1 -> Add1/2  "Engine_FC_gps"
  hr/s/1 -> Product2/2
  1/Fuel Density g to m^3/1 -> Unit Conversion kg/g and gal/m3/1
  Unit Conversion kg/g and gal/m3/1 -> Engine Diagnostics Plot/7, [FC_Cumulative_gal], "Fuel Consumption, gal"/1  "FC_Cumulative_gal"
  Sets Torq=0 if Engine Speed > Max Engine Speed (Fuel Cut)/1 -> Sum/2, Product1/2  "Engine_Torque_Nm"
  Constant1/1 -> Sum/1
  Constant2/1 -> Sets Minimum Engine Speed if Engine Speed > Min Engine Speed/3
  [Engine_FC_gps] -> Bus Creator/4  "Engine_FC_gps"
  [FC_Cumulative_gal] -> Bus Creator/5  "FC_Cumulative_gal"
  Engine Stop 0 = Normal Opt 1 = Stops Engine/1 -> Logical Operator/1
  Sets Minimum Engine Speed if Engine Speed > Min Engine Speed/1 -> Product3/2
  Logical Operator/1 -> Data Type Conversion/1
  Product3/1 -> [Engine_Speed_Actual_rpm]
  Product4/1 -> [Engine_Torque_Nm], "Engine Torque, Nm"/1, Engine Diagnostics Plot/3  "Engine_Torque_Nm"
  [Engine_Run] -> Product4/1
  Sum/1 -> Product4/2  "Engine_Torque_Net_Nm"
  Product5/1 -> [Engine_Torque_Request]
  Normalized Engine Torque Request/1 -> Product5/2
  [Engine_Run] -> Product5/1
  Data Type Conversion/1 -> Transfer Fcn/1
  [Engine_Run] -> Compare To c1/1
  Integer Delay/1 -> Add/2
  Constant3/1 -> Product6/2
  Product6/1 -> Add1/1, Scope/4
  Add1/1 -> Integrator/1, [Engine_FC_gps], Engine Diagnostics Plot/6  "Engine_FC_gps"
  Integrator/1 -> 1/Fuel Density g to m^3/1  "grams of fuel"
  Transfer Fcn/1 -> Product3/1, [Engine_Run]
  Data Type Conversion1/1 -> Product6/1, Scope/3
  Compare To Constant1/1 -> Data Type Conversion1/1
  Add/1 -> Compare To Constant1/1, Scope/2
  Compare To c1/1 -> Data Type Conversion3/1
  Data Type Conversion3/1 -> Add/1, Scope/1, Integer Delay/1
  Aux. load driven by alternator/1 -> hr/s1/1
  hr/s1/1 -> Product7/1
  [Engine_BSFC_gkWh] -> hr/s2/1
  hr/s2/1 -> Product7/2
  Switch/1 -> Add1/3
  Battery SOC/1 -> [Battery_SOC]
  [Battery_SOC] -> Switch/2
  Constant4/1 -> Switch/1
  Product7/1 -> Factor to account for  alternator and engine loses/1
  Factor to account for  alternator and engine loses/1 -> Switch/3

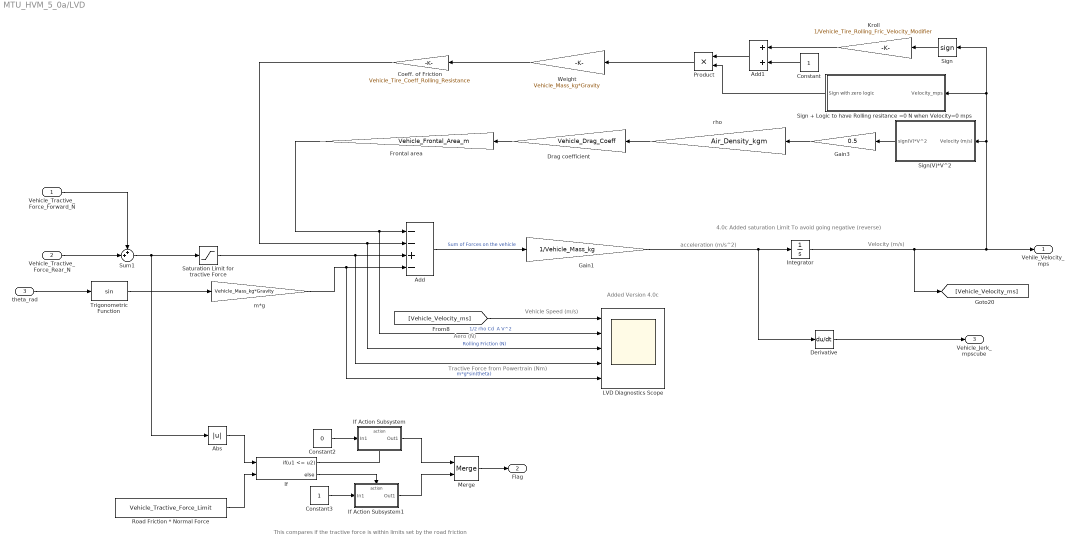
== system MTU_HVM_5_0a/LVD ==
  note: This compares if the tractive force is within limits set by the road friction
  note: acceleration (m/s^2)
  note: Velocity (m/s)
  note: Tractive Force from Powertrain (Nm)
  note: Aero (N)
  note: Vehicle Speed (m/s)
  note: 4.0c Added saturation Limit
      | To avoid going negative (reverse)
  note: Added Version 4.0c
  Vehicle_Tractive_Force_Forward_N : Inport
  Vehicle_Tractive_Force_Rear_N : Inport  Port=2
  theta_rad : Inport  Port=3
  Abs : Abs
  Add : Sum  Inputs=--+-
  Add1 : Sum
  Coeff. of Friction : Gain  Gain=Vehicle_Tire_Coeff_Rolling_Resistance
  Constant : Constant
  Constant2 : Constant  Value=0
  Constant3 : Constant
  Derivative : Derivative  LinearizePole=1
  Drag coefficient : Gain  Gain=Vehicle_Drag_Coeff
  Frontal area : Gain  Gain=Vehicle_Frontal_Area_m
  Gain1 : Gain  Gain=1/Vehicle_Mass_kg
  Gain3 : Gain  Gain=0.5
  If : If  NumInputs=2  IfExpression=u1 <= u2
  If Action Subsystem : Subsystem  TreatAsAtomicUnit=on
  If Action Subsystem1 : Subsystem  TreatAsAtomicUnit=on
  Integrator : Integrator  LimitOutput=on  LowerSaturationLimit=0
  Kroll : Gain  Gain=1/Vehicle_Tire_Rolling_Fric_Velocity_Modifier
  LVD Diagnostics Scope : Scope  NumInputPorts=5
      settings: YMin=-2~0~0~-5000~-5  YMax=2~300~150~5000~5  SaveName=Diagnostics_LVD  SampleInput=on  SampleTime=0.5
  Merge : Merge
  Product : Product  RndMeth=Zero
  Road Friction * Normal Force : Constant  Value=Vehicle_Tractive_Force_Limit
  Saturation Limit for tractive Force : Saturate  UpperLimit=Vehicle_Tractive_Force_Limit  LowerLimit=-Vehicle_Tractive_Force_Limit
  Sign : Signum  ZeroCross=off
  Sign + Logic to have Rolling resitance =0 N when Velocity=0 mps : Subsystem
  Sign(V)*V^2 : Subsystem
  Sum1 : Sum  Inputs=++|
  Trigonometric Function : Trigonometry
  Weight : Gain  Gain=Vehicle_Mass_kg*Gravity
  m*g : Gain  Gain=Vehicle_Mass_kg*Gravity
  rho : Gain  Gain=Air_Density_kgm
  Vehile_Velocity_mps : Outport
  Flag : Outport  Port=2
  Vehicle_Jerk_mpscube : Outport  Port=3
  wires:
  theta_rad/1 -> Trigonometric Function/1
  Add/1 -> Gain1/1  "Sum of Forces on the vehicle"
  Gain1/1 -> Integrator/1, Derivative/1
  Integrator/1 -> Sign(V)*V^2/1(Velocity (m/s)), Sign + Logic to have Rolling resitance =0 N when Velocity=0 mps/1(Velocity_mps), Sign/1, Vehile_Velocity_mps/1, [Vehicle_Velocity_ms]
  Trigonometric Function/1 -> m*g/1
  Gain3/1 -> rho/1
  rho/1 -> Drag coefficient/1
  Frontal area/1 -> Add/1, LVD Diagnostics Scope/2  "1/2 rho Cd  A V^2"
  Vehicle_Tractive_Force_Rear_N/1 -> Sum1/2
  Vehicle_Tractive_Force_Forward_N/1 -> Sum1/1
  m*g/1 -> Add/4, LVD Diagnostics Scope/5  "m*g*sin(theta)"
  Sum1/1 -> Saturation Limit for tractive Force/1, Abs/1
  Kroll/1 -> Add1/1
  Weight/1 -> Coeff. of Friction/1
  Constant/1 -> Add1/2
  Coeff. of Friction/1 -> Add/2, LVD Diagnostics Scope/3  "Rolling Friction (N)"
  Sign(V)*V^2/1(sign(V)*V^2) -> Gain3/1
  Abs/1 -> If/1
  If Action Subsystem/1(Out1) -> Merge/1
  If Action Subsystem1/1(Out1) -> Merge/2
  Merge/1 -> Flag/1
  If/1 -> If Action Subsystem/Action
  If/2 -> If Action Subsystem1/Action
  Road Friction * Normal Force/1 -> If/2
  Constant3/1 -> If Action Subsystem1/1(In1)
  Constant2/1 -> If Action Subsystem/1(In1)
  Add1/1 -> Product/1
  Product/1 -> Weight/1
  Derivative/1 -> Vehicle_Jerk_mpscube/1
  Drag coefficient/1 -> Frontal area/1
  Sign + Logic to have Rolling resitance =0 N when Velocity=0 mps/1(Sign with zero logic) -> Product/2
  Sign/1 -> Kroll/1
  [Vehicle_Velocity_ms] -> LVD Diagnostics Scope/1
  Saturation Limit for tractive Force/1 -> Add/3, LVD Diagnostics Scope/4

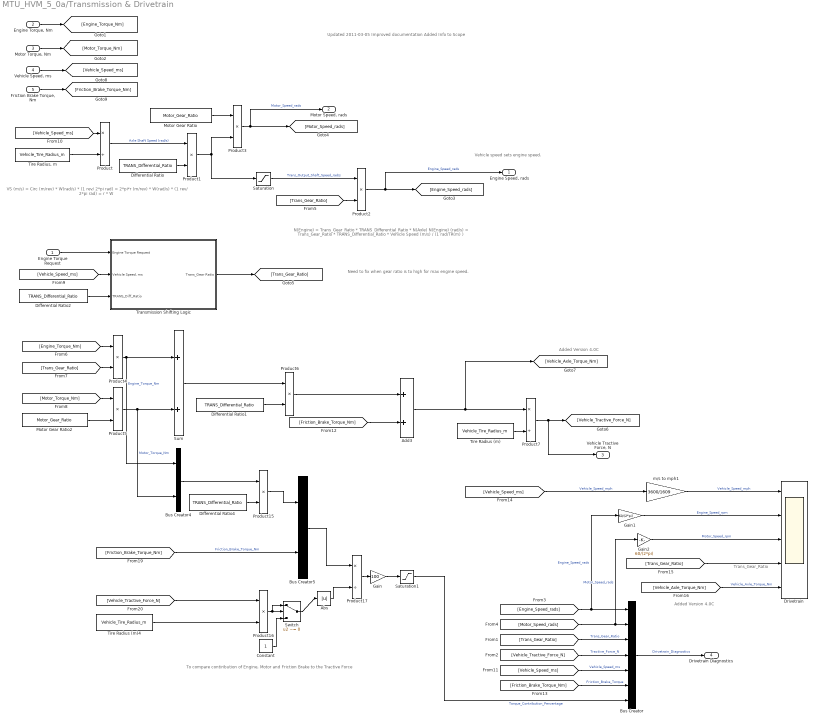
== system MTU_HVM_5_0a/Transmission & Drivetrain ==
  note: To compare contiribution of Engine, Motor and Friction Brake to the Tractive Force
  note: N(Engine) = Trans_Gear_Ratio * TRANS_Differential_Ratio * N(Axle)
      |
      | N(Engine) (rad/s) =  Trans_Gear_Ratio * TRANS_Differential_Ratio * Vehicle Speed (m/s) / (1 rad/TR(m) )
  note: VS (m/s) = Circ (m/rev) * W(rad/s) * (1 rev/ 2*pi rad)
      | = 2*pi*r (m/rev) * W(rad/s) * (1 rev/ 2*pi rad)
      | = r * W
  note: Vehicle speed sets
      | engine speed.
  note: Updated 2011-03-05
      | Improved documentation
      | Added Info to Scope
  note: Need to fix when gear ratio is to high for max engine speed.
  note: Added Version 4.0C
  note: Added Version 4.0C
  note: Trans_Gear_Ratio
  Engine Torque Request : Inport
  "Engine Torque, Nm" : Inport  Port=2
  "Motor Torque, Nm" : Inport  Port=3
  "Vehicle Speed, ms" : Inport  Port=4
  "Friction Brake Torque, Nm" : Inport  Port=5
  Abs : Abs
  Add3 : Sum
  Bus Creator : BusCreator  Inputs=7
  Bus Creator4 : BusCreator  Inputs=2
  Bus Creator5 : BusCreator  Inputs=2
  Constant : Constant
  Differential Ratio{,1..2,4} (4 alike) : Constant  Value=TRANS_Differential_Ratio
  Drivetrain : Scope  NumInputPorts=5
      settings: TimeRange=1000  YMin=0~-5000~-5~-5~-5  YMax=3000~5000~5~5~5  SaveName=Diagnostics_Drivetrain  SampleInput=on  SampleTime=0.1
  Gain : Gain  Gain=100
  Gain1 : Gain  Gain=60/(2*pi)
  Gain2 : Gain  Gain=60/(2*pi)
  Motor Gear Ratio : Constant  Value=Motor_Gear_Ratio
  Motor Gear Ratio2 : Constant  Value=Motor_Gear_Ratio
  Product : Product  Inputs=*/  RndMeth=Zero
  Product{1..6,15..16} (8 alike) : Product  RndMeth=Zero
  Product17 : Product  Inputs=*/  RndMeth=Zero
  Product7 : Product  Inputs=*/  RndMeth=Zero
  Saturation : Saturate  UpperLimit=inf  LowerLimit=0
  Saturation1 : Saturate  UpperLimit=100  LowerLimit=-100
  Sum : Sum
  Switch : Switch  Criteria=u2 ~= 0
  Tire Radius (m) : Constant  Value=Vehicle_Tire_Radius_m
  Tire Radius (m)4 : Constant  Value=Vehicle_Tire_Radius_m
  "Tire Radius, m" : Constant  Value=Vehicle_Tire_Radius_m
  Transmission Shifting Logic : Subsystem
  m/s to mph1 : Gain  Gain=3600/1609
  "Engine Speed, rads" : Outport
  "Motor Speed, rads" : Outport  Port=2
  "Vehicle Tractive Force, N" : Outport  Port=3
  Drivetrain Diagnostics : Outport  Port=4
  wires:
  Bus Creator/1 -> Drivetrain Diagnostics/1  "Drivetrain_Diagnostics"
  "Tire Radius, m"/1 -> Product/2
  Differential Ratio/1 -> Product1/2
  Product/1 -> Product1/1  "Axle Shaft Speed (rad/s)"
  Product2/1 -> [Engine_Speed_rads], "Engine Speed, rads"/1  "Engine_Speed_rads"
  Motor Gear Ratio/1 -> Product3/1
  Product3/1 -> [Motor_Speed_rads], "Motor Speed, rads"/1  "Motor_Speed_rads"
  [Trans_Gear_Ratio] -> Product2/2
  Product1/1 -> Product3/2, Saturation/1
  [Trans_Gear_Ratio] -> Bus Creator/3  "Trans_Gear_Ratio"
  [Vehicle_Tractive_Force_N] -> Bus Creator/4  "Tractive_Force_N"
  [Engine_Speed_rads] -> Bus Creator/1, Gain1/1  "Engine_Speed_rads"
  [Motor_Speed_rads] -> Bus Creator/2, Gain2/1  "Motor_Speed_rads"
  "Engine Torque, Nm"/1 -> [Engine_Torque_Nm]
  "Motor Torque, Nm"/1 -> [Motor_Torque_Nm]
  Transmission Shifting Logic/1(Trans_Gear Ratio) -> [Trans_Gear_Ratio]
  "Vehicle Speed, ms"/1 -> [Vehicle_Speed_ms]
  Engine Torque Request/1 -> Transmission Shifting Logic/1(Engine Torque Request)
  [Motor_Torque_Nm] -> Product5/1
  Motor Gear Ratio2/1 -> Product5/2
  Product5/1 -> Sum/2, Bus Creator4/2  "Motor_Torque_Nm"
  Product4/1 -> Sum/1, Bus Creator4/1  "Engine_Torque_Nm"
  Product7/1 -> [Vehicle_Tractive_Force_N], "Vehicle Tractive Force, N"/1
  [Engine_Torque_Nm] -> Product4/1
  Sum/1 -> Product6/1
  Differential Ratio1/1 -> Product6/2
  Tire Radius (m)/1 -> Product7/2
  [Trans_Gear_Ratio] -> Product4/2
  [Vehicle_Speed_ms] -> Transmission Shifting Logic/2("Vehicle Speed, ms")
  [Vehicle_Speed_ms] -> Product/1
  [Vehicle_Speed_ms] -> Bus Creator/5  "Vehicle_Speed_ms"
  "Friction Brake Torque, Nm"/1 -> [Friction_Brake_Torque_Nm]
  Product6/1 -> Add3/1
  [Friction_Brake_Torque_Nm] -> Add3/2
  Add3/1 -> Product7/1, [Vehicle_Axle_Torque_Nm]
  [Friction_Brake_Torque_Nm] -> Bus Creator/6  "Friction_Brake_Torque"
  Differential Ratio4/1 -> Product15/2
  Bus Creator4/1 -> Product15/1
  [Friction_Brake_Torque_Nm] -> Bus Creator5/2  "Friction_Brake_Torque_Nm"
  Product15/1 -> Bus Creator5/1
  [Vehicle_Tractive_Force_N] -> Product16/1
  Tire Radius (m)4/1 -> Product16/2
  Bus Creator5/1 -> Product17/1
  Saturation/1 -> Product2/1  "Trans_Output_Shaft_Speed_rad/s"
  Product17/1 -> Gain/1
  Gain/1 -> Saturation1/1
  Saturation1/1 -> Bus Creator/7  "Torque_Contribution_Percentage"
  Product16/1 -> Switch/2, Switch/1
  Switch/1 -> Abs/1
  Constant/1 -> Switch/3
  Abs/1 -> Product17/2
  Gain1/1 -> Drivetrain/2  "Engine_Speed_rpm"
  Gain2/1 -> Drivetrain/3  "Motor_Speed_rpm"
  Differential Ratio2/1 -> Transmission Shifting Logic/3(TRANS_Diff_Ratio)
  [Vehicle_Speed_ms] -> m/s to mph1/1  "Vehicle_Speed_mph"
  [Trans_Gear_Ratio] -> Drivetrain/4
  m/s to mph1/1 -> Drivetrain/1  "Vehicle_Speed_mph"
  [Vehicle_Axle_Torque_Nm] -> Drivetrain/5  "Vehicle_Axle_Torque_Nm"

== system MTU_HVM_5_0a/Vehicle Diagnostics (See Scope in here) ==
  Vehicle Bus In : Inport
  Bus Selector : BusSelector  OutputSignals=Driver_Diagnostics.Driver_Target_Speed_mph,Driver_Diagnostics.Vehicle_Speed_mph,Engine_Diagnostics.Engine_Torque_Nm,Motor_Diagnostics.Motor_Torque_Nm,Drivetrain_Diagnostics.Friction_Brake_Torque,Drivetrain_Diagnostics.Tractive_Force_N,Drivetrain_Diagnostics.Torque_Contribution_Percentage,Battery_Diagnostics.Battery_SOC,Engine_Diagnostics.Engine_FC_gps,Driver_Diagnostics.Vehicle_Jerk_mpscube
  Diagnostics : Scope  NumInputPorts=9
      settings: TimeRange=600  YMin=0~0~-1~-2000~-5000~-100~0~-5~-1  YMax=100~400~1~0~5000~100~1~5~1.75  SaveName=Diagnostics  SampleInput=on  SampleTime=0.1
  Mux : Mux  Inputs=2
  wires:
  Vehicle Bus In/1 -> Bus Selector/1
  Bus Selector/1 -> Mux/1  "<Driver_Target_Speed_mph>"
  Mux/1 -> Diagnostics/1
  Bus Selector/2 -> Mux/2  "<Vehicle_Speed_mph>"
  Bus Selector/3 -> Diagnostics/2  "<Engine_Torque_Nm>"
  Bus Selector/4 -> Diagnostics/3  "<Motor_Torque_Nm>"
  Bus Selector/5 -> Diagnostics/4  "<Friction_Brake_Torque>"
  Bus Selector/6 -> Diagnostics/5  "<Tractive_Force_N>"
  Bus Selector/7 -> Diagnostics/6  "<Torque_Contribution_Percentage>"
  Bus Selector/8 -> Diagnostics/7  "<Battery_SOC>"
  Bus Selector/9 -> Diagnostics/8  "<Engine_FC_gps>"
  Bus Selector/10 -> Diagnostics/9  "<Vehicle_Jerk_mpscube>"

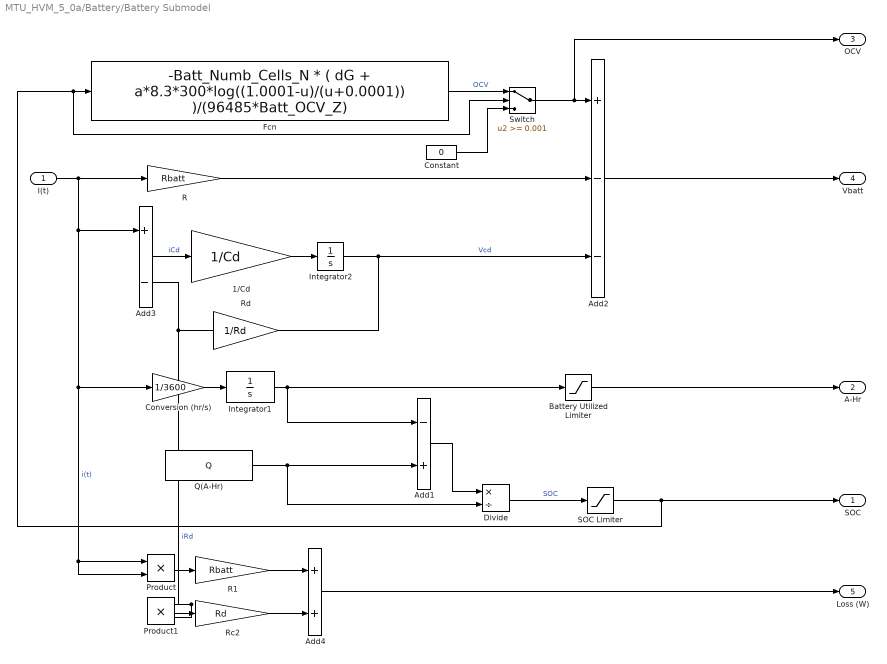
== system MTU_HVM_5_0a/Battery/Battery Submodel ==
  I(t) : Inport
  1/Cd : Gain  Gain=1/Cd
  Add1 : Sum  Inputs=-+
  Add2 : Sum  Inputs=+--
  Add3 : Sum  Inputs=+-
  Add4 : Sum
  Battery Utilized Limiter : Saturate  UpperLimit=Q*(1-Batt_Disable_SOC)  LowerLimit=0
  Constant : Constant  Value=0
  Conversion (hr/s) : Gain  Gain=1/3600
  Divide : Product  Inputs=*/
  Fcn : Fcn  Expr=-Batt_Numb_Cells_N * ( dG + a*8.3*300*log((1.0001-u)/(u+0.0001)) )/(96485*Batt_OCV_Z)
  Integrator1 : Integrator  InitialCondition=Q*(1-SOC_Init)  LimitOutput=on  UpperSaturationLimit=Q  LowerSaturationLimit=0
  Integrator2 : Integrator  UpperSaturationLimit=0  LowerSaturationLimit=0
  Product : Product  RndMeth=Zero
  Product1 : Product  RndMeth=Zero
  Q(A-Hr) : Constant  Value=Q
  R : Gain  Gain=Rbatt
  R1 : Gain  Gain=Rbatt
  Rc2 : Gain  Gain=Rd
  Rd : Gain  Gain=1/Rd
  SOC Limiter : Saturate  UpperLimit=1  LowerLimit=Batt_Disable_SOC  ZeroCross=off
  Switch : Switch  Threshold=0.001
  SOC : Outport
  A-Hr : Outport  Port=2
  OCV : Outport  Port=3
  Vbatt : Outport  Port=4
  Loss (W) : Outport  Port=5
  wires:
  R/1 -> Add2/2
  I(t)/1 -> R/1, Conversion (hr/s)/1, Product/1, Product/2, Add3/1  "i(t)"
  Q(A-Hr)/1 -> Add1/2, Divide/2
  Add1/1 -> Divide/1
  Divide/1 -> SOC Limiter/1  "SOC"
  Conversion (hr/s)/1 -> Integrator1/1
  Integrator1/1 -> Add1/1, Battery Utilized Limiter/1
  1/Cd/1 -> Integrator2/1
  Integrator2/1 -> Rd/1, Add2/3  "Vcd"
  Add3/1 -> 1/Cd/1  "iCd"
  Rd/1 -> Add3/2, Product1/1, Product1/2  "iRd"
  Product/1 -> R1/1
  Product1/1 -> Rc2/1
  R1/1 -> Add4/1
  Rc2/1 -> Add4/2
  Add4/1 -> Loss (W)/1
  Fcn/1 -> Switch/1  "OCV"
  Constant/1 -> Switch/3
  Switch/1 -> Add2/1, OCV/1
  Add2/1 -> Vbatt/1
  SOC Limiter/1 -> Fcn/1, Switch/2, SOC/1
  Battery Utilized Limiter/1 -> A-Hr/1

== system MTU_HVM_5_0a/Driver/Driver Feedback Control ==
  note: CHANGE gains for
      | Driver Control
  Target_Speed_mph : Inport
  Vehicle_Speed_mph : Inport  Port=2
  -1 to 1 : Saturate  UpperLimit=1  LowerLimit=-1
  Integral Gain : Gain  Gain=0.025
  Integrator : Integrator  ExternalReset=falling  LimitOutput=on  UpperSaturationLimit=25  LowerSaturationLimit=-25
  Sum : Sum  Inputs=|+-
  Sum1 : Sum  Inputs=++|
  Throttle Gain : Gain  Gain=0.1
  Vehicle Speed Controller : Scope  NumInputPorts=3
      settings: YMin=-0.1~-0.15~-0.1  YMax=0.7~0.35~0.8  SaveName=ScopeData3  SampleInput=on  SampleTime=0.1
  Vehicle_Speed_Error_mph : Outport
  Torque_Request_Normalized : Outport  Port=2
  wires:
  Vehicle_Speed_mph/1 -> Integrator/2, Sum/2
  Integrator/1 -> Integral Gain/1
  Integral Gain/1 -> Sum1/1, Vehicle Speed Controller/1  "Integral Term"
  Sum/1 -> Throttle Gain/1, Integrator/1, Vehicle_Speed_Error_mph/1  "Vehicle_Speed_Error_mph"
  Throttle Gain/1 -> Sum1/2, Vehicle Speed Controller/2  "Proportional Term"
  Sum1/1 -> -1 to 1/1, Vehicle Speed Controller/3  "Total Control"
  -1 to 1/1 -> Torque_Request_Normalized/1
  Target_Speed_mph/1 -> Sum/1

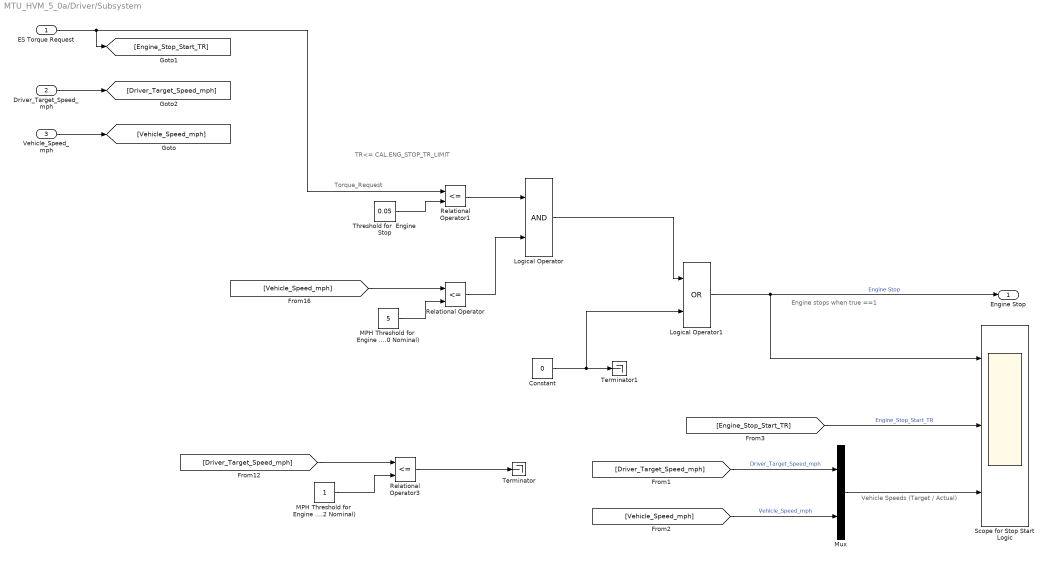
== system MTU_HVM_5_0a/Driver/Subsystem ==
  note: Engine stops when
      |
      | true ==1
  note: Torque_Request
  note: Vehicle Speeds (Target / Actual)
  note: TR<= CAL.ENG_STOP_TR_LIMIT
  ES Torque Request : Inport
  Driver_Target_Speed_mph : Inport  Port=2
  Vehicle_Speed_mph : Inport  Port=3
  Constant : Constant  Value=0  OutDataTypeStr=boolean
  Logical Operator : Logic  AllPortsSameDT=off  OutDataTypeStr=boolean
  Logical Operator1 : Logic  Operator=OR  AllPortsSameDT=off  OutDataTypeStr=boolean
  MPH Threshold for  Engine Stop (0.2 Nominal) : Constant
  MPH Threshold for  Engine Stop When stoping (5.0 Nominal) : Constant  Value=5
  Mux : Mux  Inputs=2
  Relational Operator : RelationalOperator  Operator=<=  OutDataTypeStr=boolean
  Relational Operator1 : RelationalOperator  Operator=<=  OutDataTypeStr=boolean
  Relational Operator3 : RelationalOperator  Operator=<=  OutDataTypeStr=boolean
  Scope for Stop Start Logic : Scope  NumInputPorts=3
      settings: Description=Scope for Engine Stop-Start Logic  TimeRange=1400  YMin=-0.2~-0.5~0  YMax=1.2~0.7~60  SampleInput=on  SampleTime=0.1
  Terminator : Terminator
  Terminator1 : Terminator
  Threshold for  Engine Stop : Constant  Value=0.05
  Engine Stop : Outport
  wires:
  Threshold for  Engine Stop/1 -> Relational Operator1/2
  [Vehicle_Speed_mph] -> Relational Operator/1
  MPH Threshold for  Engine Stop When stoping (5.0 Nominal)/1 -> Relational Operator/2
  Relational Operator/1 -> Logical Operator/2
  Relational Operator1/1 -> Logical Operator/1
  Logical Operator/1 -> Logical Operator1/1
  Logical Operator1/1 -> Scope for Stop Start Logic/1, Engine Stop/1  "Engine Stop"
  ES Torque Request/1 -> Relational Operator1/1, [Engine_Stop_Start_TR]
  Driver_Target_Speed_mph/1 -> [Driver_Target_Speed_mph]
  Vehicle_Speed_mph/1 -> [Vehicle_Speed_mph]
  [Driver_Target_Speed_mph] -> Mux/1  "Driver_Target_Speed_mph"
  [Vehicle_Speed_mph] -> Mux/2  "Vehicle_Speed_mph"
  Mux/1 -> Scope for Stop Start Logic/3
  [Engine_Stop_Start_TR] -> Scope for Stop Start Logic/2  "Engine_Stop_Start_TR"
  [Driver_Target_Speed_mph] -> Relational Operator3/1
  MPH Threshold for  Engine Stop (0.2 Nominal)/1 -> Relational Operator3/2
  Relational Operator3/1 -> Terminator/1
  Constant/1 -> Terminator1/1, Logical Operator1/2

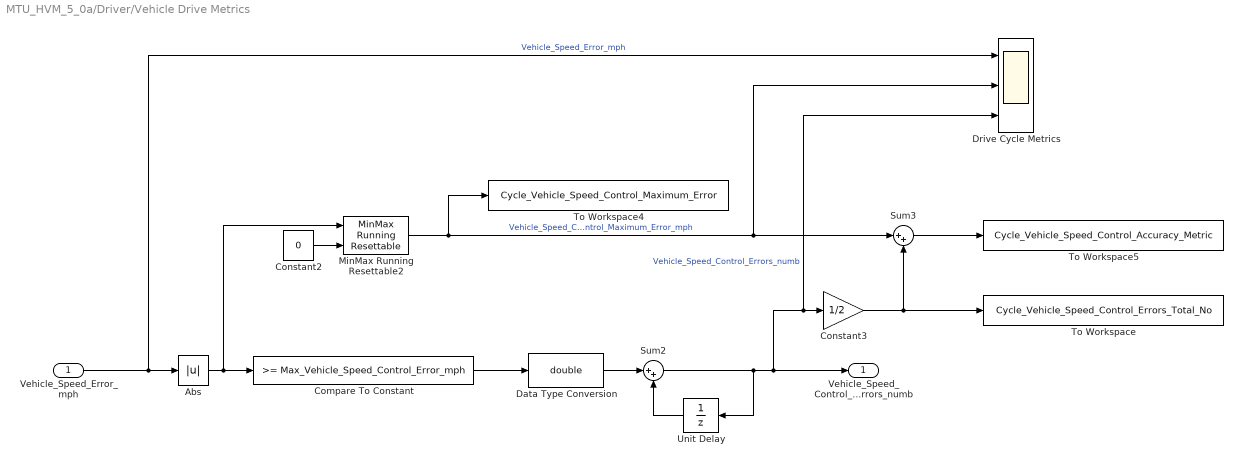
== system MTU_HVM_5_0a/Driver/Vehicle Drive Metrics ==
  Vehicle_Speed_Error_mph : Inport
  Abs : Abs
  Compare To Constant : simulink/Logic and Bit Operations/Compare To Constant  SystemSampleTime=-1  relop=>=  const=Max_Vehicle_Speed_Control_Error_mph  LogicOutDataTypeMode=boolean  ZeroCross=off
  Constant2 : Constant  Value=0
  Constant3 : Gain  Gain=1/2
  Data Type Conversion : DataTypeConversion  OutDataTypeStr=double
  Drive Cycle Metrics : Scope  NumInputPorts=3
      settings: YMin=0.2~1.65246~-1  YMax=1.1~1.8264~1  SaveName=Diagnostics_Drive_Cycle_Metrics  SampleInput=on  SampleTime=0.1
  MinMax Running Resettable2 : simulink/Math Operations/MinMax Running Resettable  SystemSampleTime=-1  Function=max  vinit=0
  Sum2 : Sum  Inputs=|++
  Sum3 : Sum  Inputs=|++
  To Workspace : ToWorkspace  VariableName=Cycle_Vehicle_Speed_Control_Errors_Total_No  SampleTime=-1  SaveFormat=Array
      settings: MaxDataPoints=1
  To Workspace4 : ToWorkspace  VariableName=Cycle_Vehicle_Speed_Control_Maximum_Error  SampleTime=-1  SaveFormat=Array
      settings: MaxDataPoints=1
  To Workspace5 : ToWorkspace  VariableName=Cycle_Vehicle_Speed_Control_Accuracy_Metric  SampleTime=-1  SaveFormat=Array
      settings: MaxDataPoints=1
  Unit Delay : UnitDelay
  Vehicle_Speed_Control_Errors_numb : Outport
  wires:
  Abs/1 -> Compare To Constant/1, MinMax Running Resettable2/1
  Compare To Constant/1 -> Data Type Conversion/1
  Sum2/1 -> Vehicle_Speed_Control_Errors_numb/1, Constant3/1, Drive Cycle Metrics/3, Unit Delay/1  "Vehicle_Speed_Control_Errors_numb"
  Unit Delay/1 -> Sum2/2
  MinMax Running Resettable2/1 -> To Workspace4/1, Sum3/1, Drive Cycle Metrics/2  "Vehicle_Speed_Control_Maximum_Error_mph"
  Constant2/1 -> MinMax Running Resettable2/2
  Sum3/1 -> To Workspace5/1
  Constant3/1 -> To Workspace/1, Sum3/2
  Data Type Conversion/1 -> Sum2/1
  Vehicle_Speed_Error_mph/1 -> Abs/1, Drive Cycle Metrics/1  "Vehicle_Speed_Error_mph"

== system MTU_HVM_5_0a/Driver/Vehicle NVH Metrics ==
  In1 : Inport
  Constant : Constant  Value=0
  Constant1 : Constant  Value=0
  MinMax Running Resettable : simulink/Math Operations/MinMax Running Resettable  SystemSampleTime=-1  Function=max  vinit=0.0
  MinMax Running Resettable1 : simulink/Math Operations/MinMax Running Resettable  SystemSampleTime=-1  Function=min  vinit=0
  Out1 : Outport
  Out2 : Outport  Port=2
  wires:
  Constant/1 -> MinMax Running Resettable/2
  Constant1/1 -> MinMax Running Resettable1/2
  In1/1 -> MinMax Running Resettable/1, MinMax Running Resettable1/1
  MinMax Running Resettable/1 -> Out1/1
  MinMax Running Resettable1/1 -> Out2/1
